simulink model "simRouteA_v4_11"  (R2015a)
settings: Solver=FixedStepDiscrete  StartTime=0.0  StopTime=36000  FixedStep=1  RelTol=1e-3
PreLoadFcn:
  | loadTimetable
StopFcn:
  | postProcess
undefined symbols (not defined in the file or in its folder): setBus1IntergenTime, setBus2IntergenTime, setBus3IntergenTime, setBus4IntergenTime
(part 7 of 7)

== system simRouteA_v4_11/atStopS18/calcPaxActivThisStop/Atomic Subsystem ==
  maxCap : Inport
  vacancy : Inport  Port=2
  paxAlight : Inport  Port=3
  paxArr : Inport  Port=4
  sec2Brd : Inport  Port=5
  Add : Sum
  Add1 : Sum
  Add2 : Sum
  Initial Value : InitialValue  Commented=on  InitialValue=0
  Min1 : MinMax  Inputs=2
  Min2 : MinMax  Inputs=2
  Product : Product
  Signal Latch : SignalLatch  Commented=on  MemoryWriteEdgeOption=Either  MemoryReadEdgeOption=Either  SpecifyReadEventPriority=on
      settings: InputPortMap=u0,u1,u2  OutputPortMap=o2
  Subtract : Sum  Inputs=+-
  Subtract1 : Sum  Inputs=-+
  Subtract2 : Sum  Inputs=+-
  Unit Delay : UnitDelay  SampleTime=-1
  newVacancy : Outport
  paxBoard : Outport  Port=2
  paxRemain : Outport  Port=3
  paxWait : Outport  Port=4
  dwellTime : Outport  Port=5
  corrPaxAlight : Outport  Port=6
  wires:
  Add/1 -> Min1/1, Subtract/1
  Min1/1 -> Subtract1/1, Subtract/2, Add2/1, paxBoard/1
  paxArr/1 -> Add1/1
  Add1/1 -> paxWait/1, Subtract1/2, Min1/2
  Subtract1/1 -> Unit Delay/1, paxRemain/1
  Unit Delay/1 -> Add1/2
  vacancy/1 -> Subtract2/2, Add/1
  maxCap/1 -> Subtract2/1
  Subtract/1 -> newVacancy/1
  Add2/1 -> Product/1
  sec2Brd/1 -> Product/2
  Product/1 -> dwellTime/1
  Subtract2/1 -> Min2/1
  Min2/1 -> corrPaxAlight/1, Add2/2, Add/2
  paxAlight/1 -> Min2/2

== system simRouteA_v4_11/atStopS18/calcPaxActivThisStop/calcPaxAlightS1 ==
  integrPax : Inport
  Subtract : Sum  Inputs=+-
  Unit Delay : UnitDelay  SampleTime=-1
  truPax : Outport
  intgPax : Outport  Port=2
  wires:
  integrPax/1 -> Unit Delay/1, intgPax/1, Subtract/1
  Subtract/1 -> truPax/1
  Unit Delay/1 -> Subtract/2

== system simRouteA_v4_11/atStopS18/calcPaxActivThisStop/calcPaxArrS1 ==
  integrPax : Inport
  Subtract : Sum  Inputs=+-
  Unit Delay : UnitDelay  SampleTime=-1
  truPax : Outport
  intgPax : Outport  Port=2
  wires:
  integrPax/1 -> Unit Delay/1, intgPax/1, Subtract/1
  Subtract/1 -> truPax/1
  Unit Delay/1 -> Subtract/2

== system simRouteA_v4_11/atStopS18/integrPaxAlightS1/Atomic Subsystem1 ==
  In1 : Inport
  Add : Sum
  Unit Delay : UnitDelay  SampleTime=-1
  Out1 : Outport
  wires:
  In1/1 -> Add/1
  Add/1 -> Out1/1, Unit Delay/1
  Unit Delay/1 -> Add/2

== system simRouteA_v4_11/atStopS18/integrPaxArrS1/Atomic Subsystem1 ==
  In1 : Inport
  Add : Sum
  Unit Delay : UnitDelay  SampleTime=-1
  Out1 : Outport
  wires:
  In1/1 -> Add/1
  Add/1 -> Out1/1, Unit Delay/1
  Unit Delay/1 -> Add/2

== system simRouteA_v4_11/atStopS2/busDwellThisStop/Subsystem2 ==
  dwellTime : Inport
  tStartSrvPax : Inport  Port=2
  Add1 : Sum
  Add2 : Sum
  Subtract : Sum  Inputs=+-
  Subtract1 : Sum  Inputs=+-
  Switch : Switch  Criteria=u2 > Threshold
  Unit Delay : UnitDelay  SampleTime=-1
  headWay : Constant  Value=3
  dwellTimeNew : Outport
  wires:
  Subtract/1 -> Switch/2
  Switch/1 -> Subtract1/1, Unit Delay/1
  headWay/1 -> Add2/1
  tStartSrvPax/1 -> Subtract1/2, Add1/2
  Add2/1 -> Switch/3
  dwellTime/1 -> Add1/1
  Subtract1/1 -> dwellTimeNew/1
  Add1/1 -> Switch/1, Subtract/1
  Unit Delay/1 -> Add2/2, Subtract/2

== system simRouteA_v4_11/atStopS2/calcPaxActivThisStop/Atomic Subsystem ==
  maxCap : Inport
  vacancy : Inport  Port=2
  paxAlight : Inport  Port=3
  paxArr : Inport  Port=4
  sec2Brd : Inport  Port=5
  Add : Sum
  Add1 : Sum
  Add2 : Sum
  Initial Value : InitialValue  Commented=on  InitialValue=0
  Min1 : MinMax  Inputs=2
  Min2 : MinMax  Inputs=2
  Product : Product
  Signal Latch : SignalLatch  Commented=on  MemoryWriteEdgeOption=Either  MemoryReadEdgeOption=Either  SpecifyReadEventPriority=on
      settings: InputPortMap=u0,u1,u2  OutputPortMap=o2
  Subtract : Sum  Inputs=+-
  Subtract1 : Sum  Inputs=-+
  Subtract2 : Sum  Inputs=+-
  Unit Delay : UnitDelay  SampleTime=-1
  newVacancy : Outport
  paxBoard : Outport  Port=2
  paxRemain : Outport  Port=3
  paxWait : Outport  Port=4
  dwellTime : Outport  Port=5
  corrPaxAlight : Outport  Port=6
  wires:
  Add/1 -> Min1/1, Subtract/1
  Min1/1 -> Subtract1/1, Subtract/2, Add2/1, paxBoard/1
  paxArr/1 -> Add1/1
  Add1/1 -> paxWait/1, Subtract1/2, Min1/2
  Subtract1/1 -> Unit Delay/1, paxRemain/1
  Unit Delay/1 -> Add1/2
  vacancy/1 -> Subtract2/2, Add/1
  maxCap/1 -> Subtract2/1
  Subtract/1 -> newVacancy/1
  Add2/1 -> Product/1
  sec2Brd/1 -> Product/2
  Product/1 -> dwellTime/1
  Subtract2/1 -> Min2/1
  Min2/1 -> corrPaxAlight/1, Add2/2, Add/2
  paxAlight/1 -> Min2/2

== system simRouteA_v4_11/atStopS2/calcPaxActivThisStop/calcPaxAlightS1 ==
  integrPax : Inport
  Subtract : Sum  Inputs=+-
  Unit Delay : UnitDelay  SampleTime=-1
  truPax : Outport
  intgPax : Outport  Port=2
  wires:
  integrPax/1 -> Unit Delay/1, intgPax/1, Subtract/1
  Subtract/1 -> truPax/1
  Unit Delay/1 -> Subtract/2

== system simRouteA_v4_11/atStopS2/calcPaxActivThisStop/calcPaxArrS1 ==
  integrPax : Inport
  Subtract : Sum  Inputs=+-
  Unit Delay : UnitDelay  SampleTime=-1
  truPax : Outport
  intgPax : Outport  Port=2
  wires:
  integrPax/1 -> Unit Delay/1, intgPax/1, Subtract/1
  Subtract/1 -> truPax/1
  Unit Delay/1 -> Subtract/2

== system simRouteA_v4_11/atStopS2/integrPaxAlightS1/Atomic Subsystem1 ==
  In1 : Inport
  Add : Sum
  Unit Delay : UnitDelay  SampleTime=-1
  Out1 : Outport
  wires:
  In1/1 -> Add/1
  Add/1 -> Out1/1, Unit Delay/1
  Unit Delay/1 -> Add/2

== system simRouteA_v4_11/atStopS2/integrPaxArrS1/Atomic Subsystem1 ==
  In1 : Inport
  Add : Sum
  Unit Delay : UnitDelay  SampleTime=-1
  Out1 : Outport
  wires:
  In1/1 -> Add/1
  Add/1 -> Out1/1, Unit Delay/1
  Unit Delay/1 -> Add/2

== system simRouteA_v4_11/atStopS3/busDwellThisStop/Subsystem2 ==
  dwellTime : Inport
  tStartSrvPax : Inport  Port=2
  Add1 : Sum
  Add2 : Sum
  Subtract : Sum  Inputs=+-
  Subtract1 : Sum  Inputs=+-
  Switch : Switch  Criteria=u2 > Threshold
  Unit Delay : UnitDelay  SampleTime=-1
  headWay : Constant  Value=3
  dwellTimeNew : Outport
  wires:
  Subtract/1 -> Switch/2
  Switch/1 -> Subtract1/1, Unit Delay/1
  headWay/1 -> Add2/1
  tStartSrvPax/1 -> Subtract1/2, Add1/2
  Add2/1 -> Switch/3
  dwellTime/1 -> Add1/1
  Subtract1/1 -> dwellTimeNew/1
  Add1/1 -> Switch/1, Subtract/1
  Unit Delay/1 -> Add2/2, Subtract/2

== system simRouteA_v4_11/atStopS3/calcPaxActivThisStop/Atomic Subsystem ==
  maxCap : Inport
  vacancy : Inport  Port=2
  paxAlight : Inport  Port=3
  paxArr : Inport  Port=4
  sec2Brd : Inport  Port=5
  Add : Sum
  Add1 : Sum
  Add2 : Sum
  Initial Value : InitialValue  Commented=on  InitialValue=0
  Min1 : MinMax  Inputs=2
  Min2 : MinMax  Inputs=2
  Product : Product
  Signal Latch : SignalLatch  Commented=on  MemoryWriteEdgeOption=Either  MemoryReadEdgeOption=Either  SpecifyReadEventPriority=on
      settings: InputPortMap=u0,u1,u2  OutputPortMap=o2
  Subtract : Sum  Inputs=+-
  Subtract1 : Sum  Inputs=-+
  Subtract2 : Sum  Inputs=+-
  Unit Delay : UnitDelay  SampleTime=-1
  newVacancy : Outport
  paxBoard : Outport  Port=2
  paxRemain : Outport  Port=3
  paxWait : Outport  Port=4
  dwellTime : Outport  Port=5
  corrPaxAlight : Outport  Port=6
  wires:
  Add/1 -> Min1/1, Subtract/1
  Min1/1 -> Subtract1/1, Subtract/2, Add2/1, paxBoard/1
  paxArr/1 -> Add1/1
  Add1/1 -> paxWait/1, Subtract1/2, Min1/2
  Subtract1/1 -> Unit Delay/1, paxRemain/1
  Unit Delay/1 -> Add1/2
  vacancy/1 -> Subtract2/2, Add/1
  maxCap/1 -> Subtract2/1
  Subtract/1 -> newVacancy/1
  Add2/1 -> Product/1
  sec2Brd/1 -> Product/2
  Product/1 -> dwellTime/1
  Subtract2/1 -> Min2/1
  Min2/1 -> corrPaxAlight/1, Add2/2, Add/2
  paxAlight/1 -> Min2/2

== system simRouteA_v4_11/atStopS3/calcPaxActivThisStop/calcPaxAlightS1 ==
  integrPax : Inport
  Subtract : Sum  Inputs=+-
  Unit Delay : UnitDelay  SampleTime=-1
  truPax : Outport
  intgPax : Outport  Port=2
  wires:
  integrPax/1 -> Unit Delay/1, intgPax/1, Subtract/1
  Subtract/1 -> truPax/1
  Unit Delay/1 -> Subtract/2

== system simRouteA_v4_11/atStopS3/calcPaxActivThisStop/calcPaxArrS1 ==
  integrPax : Inport
  Subtract : Sum  Inputs=+-
  Unit Delay : UnitDelay  SampleTime=-1
  truPax : Outport
  intgPax : Outport  Port=2
  wires:
  integrPax/1 -> Unit Delay/1, intgPax/1, Subtract/1
  Subtract/1 -> truPax/1
  Unit Delay/1 -> Subtract/2

== system simRouteA_v4_11/atStopS3/integrPaxAlightS1/Atomic Subsystem1 ==
  In1 : Inport
  Add : Sum
  Unit Delay : UnitDelay  SampleTime=-1
  Out1 : Outport
  wires:
  In1/1 -> Add/1
  Add/1 -> Out1/1, Unit Delay/1
  Unit Delay/1 -> Add/2

== system simRouteA_v4_11/atStopS3/integrPaxArrS1/Atomic Subsystem1 ==
  In1 : Inport
  Add : Sum
  Unit Delay : UnitDelay  SampleTime=-1
  Out1 : Outport
  wires:
  In1/1 -> Add/1
  Add/1 -> Out1/1, Unit Delay/1
  Unit Delay/1 -> Add/2

== system simRouteA_v4_11/atStopS4/busDwellThisStop/Subsystem2 ==
  dwellTime : Inport
  tStartSrvPax : Inport  Port=2
  Add1 : Sum
  Add2 : Sum
  Subtract : Sum  Inputs=+-
  Subtract1 : Sum  Inputs=+-
  Switch : Switch  Criteria=u2 > Threshold
  Unit Delay : UnitDelay  SampleTime=-1
  headWay : Constant  Value=3
  dwellTimeNew : Outport
  wires:
  Subtract/1 -> Switch/2
  Switch/1 -> Subtract1/1, Unit Delay/1
  headWay/1 -> Add2/1
  tStartSrvPax/1 -> Subtract1/2, Add1/2
  Add2/1 -> Switch/3
  dwellTime/1 -> Add1/1
  Subtract1/1 -> dwellTimeNew/1
  Add1/1 -> Switch/1, Subtract/1
  Unit Delay/1 -> Add2/2, Subtract/2

== system simRouteA_v4_11/atStopS4/calcPaxActivThisStop/Atomic Subsystem ==
  maxCap : Inport
  vacancy : Inport  Port=2
  paxAlight : Inport  Port=3
  paxArr : Inport  Port=4
  sec2Brd : Inport  Port=5
  Add : Sum
  Add1 : Sum
  Add2 : Sum
  Initial Value : InitialValue  Commented=on  InitialValue=0
  Min1 : MinMax  Inputs=2
  Min2 : MinMax  Inputs=2
  Product : Product
  Signal Latch : SignalLatch  Commented=on  MemoryWriteEdgeOption=Either  MemoryReadEdgeOption=Either  SpecifyReadEventPriority=on
      settings: InputPortMap=u0,u1,u2  OutputPortMap=o2
  Subtract : Sum  Inputs=+-
  Subtract1 : Sum  Inputs=-+
  Subtract2 : Sum  Inputs=+-
  Unit Delay : UnitDelay  SampleTime=-1
  newVacancy : Outport
  paxBoard : Outport  Port=2
  paxRemain : Outport  Port=3
  paxWait : Outport  Port=4
  dwellTime : Outport  Port=5
  corrPaxAlight : Outport  Port=6
  wires:
  Add/1 -> Min1/1, Subtract/1
  Min1/1 -> Subtract1/1, Subtract/2, Add2/1, paxBoard/1
  paxArr/1 -> Add1/1
  Add1/1 -> paxWait/1, Subtract1/2, Min1/2
  Subtract1/1 -> Unit Delay/1, paxRemain/1
  Unit Delay/1 -> Add1/2
  vacancy/1 -> Subtract2/2, Add/1
  maxCap/1 -> Subtract2/1
  Subtract/1 -> newVacancy/1
  Add2/1 -> Product/1
  sec2Brd/1 -> Product/2
  Product/1 -> dwellTime/1
  Subtract2/1 -> Min2/1
  Min2/1 -> corrPaxAlight/1, Add2/2, Add/2
  paxAlight/1 -> Min2/2

== system simRouteA_v4_11/atStopS4/calcPaxActivThisStop/calcPaxAlightS1 ==
  integrPax : Inport
  Subtract : Sum  Inputs=+-
  Unit Delay : UnitDelay  SampleTime=-1
  truPax : Outport
  intgPax : Outport  Port=2
  wires:
  integrPax/1 -> Unit Delay/1, intgPax/1, Subtract/1
  Subtract/1 -> truPax/1
  Unit Delay/1 -> Subtract/2

== system simRouteA_v4_11/atStopS4/calcPaxActivThisStop/calcPaxArrS1 ==
  integrPax : Inport
  Subtract : Sum  Inputs=+-
  Unit Delay : UnitDelay  SampleTime=-1
  truPax : Outport
  intgPax : Outport  Port=2
  wires:
  integrPax/1 -> Unit Delay/1, intgPax/1, Subtract/1
  Subtract/1 -> truPax/1
  Unit Delay/1 -> Subtract/2

== system simRouteA_v4_11/atStopS4/integrPaxAlightS1/Atomic Subsystem1 ==
  In1 : Inport
  Add : Sum
  Unit Delay : UnitDelay  SampleTime=-1
  Out1 : Outport
  wires:
  In1/1 -> Add/1
  Add/1 -> Out1/1, Unit Delay/1
  Unit Delay/1 -> Add/2

== system simRouteA_v4_11/atStopS4/integrPaxArrS1/Atomic Subsystem1 ==
  In1 : Inport
  Add : Sum
  Unit Delay : UnitDelay  SampleTime=-1
  Out1 : Outport
  wires:
  In1/1 -> Add/1
  Add/1 -> Out1/1, Unit Delay/1
  Unit Delay/1 -> Add/2

== system simRouteA_v4_11/atStopS5/busDwellThisStop/Subsystem2 ==
  dwellTime : Inport
  tStartSrvPax : Inport  Port=2
  Add1 : Sum
  Add2 : Sum
  Subtract : Sum  Inputs=+-
  Subtract1 : Sum  Inputs=+-
  Switch : Switch  Criteria=u2 > Threshold
  Unit Delay : UnitDelay  SampleTime=-1
  headWay : Constant  Value=3
  dwellTimeNew : Outport
  wires:
  Subtract/1 -> Switch/2
  Switch/1 -> Subtract1/1, Unit Delay/1
  headWay/1 -> Add2/1
  tStartSrvPax/1 -> Subtract1/2, Add1/2
  Add2/1 -> Switch/3
  dwellTime/1 -> Add1/1
  Subtract1/1 -> dwellTimeNew/1
  Add1/1 -> Switch/1, Subtract/1
  Unit Delay/1 -> Add2/2, Subtract/2

== system simRouteA_v4_11/atStopS5/calcPaxActivThisStop/Atomic Subsystem ==
  maxCap : Inport
  vacancy : Inport  Port=2
  paxAlight : Inport  Port=3
  paxArr : Inport  Port=4
  sec2Brd : Inport  Port=5
  Add : Sum
  Add1 : Sum
  Add2 : Sum
  Initial Value : InitialValue  Commented=on  InitialValue=0
  Min1 : MinMax  Inputs=2
  Min2 : MinMax  Inputs=2
  Product : Product
  Signal Latch : SignalLatch  Commented=on  MemoryWriteEdgeOption=Either  MemoryReadEdgeOption=Either  SpecifyReadEventPriority=on
      settings: InputPortMap=u0,u1,u2  OutputPortMap=o2
  Subtract : Sum  Inputs=+-
  Subtract1 : Sum  Inputs=-+
  Subtract2 : Sum  Inputs=+-
  Unit Delay : UnitDelay  SampleTime=-1
  newVacancy : Outport
  paxBoard : Outport  Port=2
  paxRemain : Outport  Port=3
  paxWait : Outport  Port=4
  dwellTime : Outport  Port=5
  corrPaxAlight : Outport  Port=6
  wires:
  Add/1 -> Min1/1, Subtract/1
  Min1/1 -> Subtract1/1, Subtract/2, Add2/1, paxBoard/1
  paxArr/1 -> Add1/1
  Add1/1 -> paxWait/1, Subtract1/2, Min1/2
  Subtract1/1 -> Unit Delay/1, paxRemain/1
  Unit Delay/1 -> Add1/2
  vacancy/1 -> Subtract2/2, Add/1
  maxCap/1 -> Subtract2/1
  Subtract/1 -> newVacancy/1
  Add2/1 -> Product/1
  sec2Brd/1 -> Product/2
  Product/1 -> dwellTime/1
  Subtract2/1 -> Min2/1
  Min2/1 -> corrPaxAlight/1, Add2/2, Add/2
  paxAlight/1 -> Min2/2

== system simRouteA_v4_11/atStopS5/calcPaxActivThisStop/calcPaxAlightS1 ==
  integrPax : Inport
  Subtract : Sum  Inputs=+-
  Unit Delay : UnitDelay  SampleTime=-1
  truPax : Outport
  intgPax : Outport  Port=2
  wires:
  integrPax/1 -> Unit Delay/1, intgPax/1, Subtract/1
  Subtract/1 -> truPax/1
  Unit Delay/1 -> Subtract/2

== system simRouteA_v4_11/atStopS5/calcPaxActivThisStop/calcPaxArrS1 ==
  integrPax : Inport
  Subtract : Sum  Inputs=+-
  Unit Delay : UnitDelay  SampleTime=-1
  truPax : Outport
  intgPax : Outport  Port=2
  wires:
  integrPax/1 -> Unit Delay/1, intgPax/1, Subtract/1
  Subtract/1 -> truPax/1
  Unit Delay/1 -> Subtract/2

== system simRouteA_v4_11/atStopS5/integrPaxAlightS1/Atomic Subsystem1 ==
  In1 : Inport
  Add : Sum
  Unit Delay : UnitDelay  SampleTime=-1
  Out1 : Outport
  wires:
  In1/1 -> Add/1
  Add/1 -> Out1/1, Unit Delay/1
  Unit Delay/1 -> Add/2

== system simRouteA_v4_11/atStopS5/integrPaxArrS1/Atomic Subsystem1 ==
  In1 : Inport
  Add : Sum
  Unit Delay : UnitDelay  SampleTime=-1
  Out1 : Outport
  wires:
  In1/1 -> Add/1
  Add/1 -> Out1/1, Unit Delay/1
  Unit Delay/1 -> Add/2

== system simRouteA_v4_11/atStopS6/busDwellThisStop/Subsystem2 ==
  dwellTime : Inport
  tStartSrvPax : Inport  Port=2
  Add1 : Sum
  Add2 : Sum
  Subtract : Sum  Inputs=+-
  Subtract1 : Sum  Inputs=+-
  Switch : Switch  Criteria=u2 > Threshold
  Unit Delay : UnitDelay  SampleTime=-1
  headWay : Constant  Value=3
  dwellTimeNew : Outport
  wires:
  Subtract/1 -> Switch/2
  Switch/1 -> Subtract1/1, Unit Delay/1
  headWay/1 -> Add2/1
  tStartSrvPax/1 -> Subtract1/2, Add1/2
  Add2/1 -> Switch/3
  dwellTime/1 -> Add1/1
  Subtract1/1 -> dwellTimeNew/1
  Add1/1 -> Switch/1, Subtract/1
  Unit Delay/1 -> Add2/2, Subtract/2

== system simRouteA_v4_11/atStopS6/calcPaxActivThisStop/Atomic Subsystem ==
  maxCap : Inport
  vacancy : Inport  Port=2
  paxAlight : Inport  Port=3
  paxArr : Inport  Port=4
  sec2Brd : Inport  Port=5
  Add : Sum
  Add1 : Sum
  Add2 : Sum
  Initial Value : InitialValue  Commented=on  InitialValue=0
  Min1 : MinMax  Inputs=2
  Min2 : MinMax  Inputs=2
  Product : Product
  Signal Latch : SignalLatch  Commented=on  MemoryWriteEdgeOption=Either  MemoryReadEdgeOption=Either  SpecifyReadEventPriority=on
      settings: InputPortMap=u0,u1,u2  OutputPortMap=o2
  Subtract : Sum  Inputs=+-
  Subtract1 : Sum  Inputs=-+
  Subtract2 : Sum  Inputs=+-
  Unit Delay : UnitDelay  SampleTime=-1
  newVacancy : Outport
  paxBoard : Outport  Port=2
  paxRemain : Outport  Port=3
  paxWait : Outport  Port=4
  dwellTime : Outport  Port=5
  corrPaxAlight : Outport  Port=6
  wires:
  Add/1 -> Min1/1, Subtract/1
  Min1/1 -> Subtract1/1, Subtract/2, Add2/1, paxBoard/1
  paxArr/1 -> Add1/1
  Add1/1 -> paxWait/1, Subtract1/2, Min1/2
  Subtract1/1 -> Unit Delay/1, paxRemain/1
  Unit Delay/1 -> Add1/2
  vacancy/1 -> Subtract2/2, Add/1
  maxCap/1 -> Subtract2/1
  Subtract/1 -> newVacancy/1
  Add2/1 -> Product/1
  sec2Brd/1 -> Product/2
  Product/1 -> dwellTime/1
  Subtract2/1 -> Min2/1
  Min2/1 -> corrPaxAlight/1, Add2/2, Add/2
  paxAlight/1 -> Min2/2

== system simRouteA_v4_11/atStopS6/calcPaxActivThisStop/calcPaxAlightS1 ==
  integrPax : Inport
  Subtract : Sum  Inputs=+-
  Unit Delay : UnitDelay  SampleTime=-1
  truPax : Outport
  intgPax : Outport  Port=2
  wires:
  integrPax/1 -> Unit Delay/1, intgPax/1, Subtract/1
  Subtract/1 -> truPax/1
  Unit Delay/1 -> Subtract/2

== system simRouteA_v4_11/atStopS6/calcPaxActivThisStop/calcPaxArrS1 ==
  integrPax : Inport
  Subtract : Sum  Inputs=+-
  Unit Delay : UnitDelay  SampleTime=-1
  truPax : Outport
  intgPax : Outport  Port=2
  wires:
  integrPax/1 -> Unit Delay/1, intgPax/1, Subtract/1
  Subtract/1 -> truPax/1
  Unit Delay/1 -> Subtract/2

== system simRouteA_v4_11/atStopS6/integrPaxAlightS1/Atomic Subsystem1 ==
  In1 : Inport
  Add : Sum
  Unit Delay : UnitDelay  SampleTime=-1
  Out1 : Outport
  wires:
  In1/1 -> Add/1
  Add/1 -> Out1/1, Unit Delay/1
  Unit Delay/1 -> Add/2

== system simRouteA_v4_11/atStopS6/integrPaxArrS1/Atomic Subsystem1 ==
  In1 : Inport
  Add : Sum
  Unit Delay : UnitDelay  SampleTime=-1
  Out1 : Outport
  wires:
  In1/1 -> Add/1
  Add/1 -> Out1/1, Unit Delay/1
  Unit Delay/1 -> Add/2

== system simRouteA_v4_11/atStopS7/busDwellThisStop/Subsystem2 ==
  dwellTime : Inport
  tStartSrvPax : Inport  Port=2
  Add1 : Sum
  Add2 : Sum
  Subtract : Sum  Inputs=+-
  Subtract1 : Sum  Inputs=+-
  Switch : Switch  Criteria=u2 > Threshold
  Unit Delay : UnitDelay  SampleTime=-1
  headWay : Constant  Value=3
  dwellTimeNew : Outport
  wires:
  Subtract/1 -> Switch/2
  Switch/1 -> Subtract1/1, Unit Delay/1
  headWay/1 -> Add2/1
  tStartSrvPax/1 -> Subtract1/2, Add1/2
  Add2/1 -> Switch/3
  dwellTime/1 -> Add1/1
  Subtract1/1 -> dwellTimeNew/1
  Add1/1 -> Switch/1, Subtract/1
  Unit Delay/1 -> Add2/2, Subtract/2

== system simRouteA_v4_11/atStopS7/calcPaxActivThisStop/Atomic Subsystem ==
  maxCap : Inport
  vacancy : Inport  Port=2
  paxAlight : Inport  Port=3
  paxArr : Inport  Port=4
  sec2Brd : Inport  Port=5
  Add : Sum
  Add1 : Sum
  Add2 : Sum
  Initial Value : InitialValue  Commented=on  InitialValue=0
  Min1 : MinMax  Inputs=2
  Min2 : MinMax  Inputs=2
  Product : Product
  Signal Latch : SignalLatch  Commented=on  MemoryWriteEdgeOption=Either  MemoryReadEdgeOption=Either  SpecifyReadEventPriority=on
      settings: InputPortMap=u0,u1,u2  OutputPortMap=o2
  Subtract : Sum  Inputs=+-
  Subtract1 : Sum  Inputs=-+
  Subtract2 : Sum  Inputs=+-
  Unit Delay : UnitDelay  SampleTime=-1
  newVacancy : Outport
  paxBoard : Outport  Port=2
  paxRemain : Outport  Port=3
  paxWait : Outport  Port=4
  dwellTime : Outport  Port=5
  corrPaxAlight : Outport  Port=6
  wires:
  Add/1 -> Min1/1, Subtract/1
  Min1/1 -> Subtract1/1, Subtract/2, Add2/1, paxBoard/1
  paxArr/1 -> Add1/1
  Add1/1 -> paxWait/1, Subtract1/2, Min1/2
  Subtract1/1 -> Unit Delay/1, paxRemain/1
  Unit Delay/1 -> Add1/2
  vacancy/1 -> Subtract2/2, Add/1
  maxCap/1 -> Subtract2/1
  Subtract/1 -> newVacancy/1
  Add2/1 -> Product/1
  sec2Brd/1 -> Product/2
  Product/1 -> dwellTime/1
  Subtract2/1 -> Min2/1
  Min2/1 -> corrPaxAlight/1, Add2/2, Add/2
  paxAlight/1 -> Min2/2

== system simRouteA_v4_11/atStopS7/calcPaxActivThisStop/calcPaxAlightS1 ==
  integrPax : Inport
  Subtract : Sum  Inputs=+-
  Unit Delay : UnitDelay  SampleTime=-1
  truPax : Outport
  intgPax : Outport  Port=2
  wires:
  integrPax/1 -> Unit Delay/1, intgPax/1, Subtract/1
  Subtract/1 -> truPax/1
  Unit Delay/1 -> Subtract/2

== system simRouteA_v4_11/atStopS7/calcPaxActivThisStop/calcPaxArrS1 ==
  integrPax : Inport
  Subtract : Sum  Inputs=+-
  Unit Delay : UnitDelay  SampleTime=-1
  truPax : Outport
  intgPax : Outport  Port=2
  wires:
  integrPax/1 -> Unit Delay/1, intgPax/1, Subtract/1
  Subtract/1 -> truPax/1
  Unit Delay/1 -> Subtract/2

== system simRouteA_v4_11/atStopS7/integrPaxAlightS1/Atomic Subsystem1 ==
  In1 : Inport
  Add : Sum
  Unit Delay : UnitDelay  SampleTime=-1
  Out1 : Outport
  wires:
  In1/1 -> Add/1
  Add/1 -> Out1/1, Unit Delay/1
  Unit Delay/1 -> Add/2

== system simRouteA_v4_11/atStopS7/integrPaxArrS1/Atomic Subsystem1 ==
  In1 : Inport
  Add : Sum
  Unit Delay : UnitDelay  SampleTime=-1
  Out1 : Outport
  wires:
  In1/1 -> Add/1
  Add/1 -> Out1/1, Unit Delay/1
  Unit Delay/1 -> Add/2

== system simRouteA_v4_11/atStopS8/busDwellThisStop/Subsystem2 ==
  dwellTime : Inport
  tStartSrvPax : Inport  Port=2
  Add1 : Sum
  Add2 : Sum
  Subtract : Sum  Inputs=+-
  Subtract1 : Sum  Inputs=+-
  Switch : Switch  Criteria=u2 > Threshold
  Unit Delay : UnitDelay  SampleTime=-1
  headWay : Constant  Value=3
  dwellTimeNew : Outport
  wires:
  Subtract/1 -> Switch/2
  Switch/1 -> Subtract1/1, Unit Delay/1
  headWay/1 -> Add2/1
  tStartSrvPax/1 -> Subtract1/2, Add1/2
  Add2/1 -> Switch/3
  dwellTime/1 -> Add1/1
  Subtract1/1 -> dwellTimeNew/1
  Add1/1 -> Switch/1, Subtract/1
  Unit Delay/1 -> Add2/2, Subtract/2

== system simRouteA_v4_11/atStopS8/calcPaxActivThisStop/Atomic Subsystem ==
  maxCap : Inport
  vacancy : Inport  Port=2
  paxAlight : Inport  Port=3
  paxArr : Inport  Port=4
  sec2Brd : Inport  Port=5
  Add : Sum
  Add1 : Sum
  Add2 : Sum
  Initial Value : InitialValue  Commented=on  InitialValue=0
  Min1 : MinMax  Inputs=2
  Min2 : MinMax  Inputs=2
  Product : Product
  Signal Latch : SignalLatch  Commented=on  MemoryWriteEdgeOption=Either  MemoryReadEdgeOption=Either  SpecifyReadEventPriority=on
      settings: InputPortMap=u0,u1,u2  OutputPortMap=o2
  Subtract : Sum  Inputs=+-
  Subtract1 : Sum  Inputs=-+
  Subtract2 : Sum  Inputs=+-
  Unit Delay : UnitDelay  SampleTime=-1
  newVacancy : Outport
  paxBoard : Outport  Port=2
  paxRemain : Outport  Port=3
  paxWait : Outport  Port=4
  dwellTime : Outport  Port=5
  corrPaxAlight : Outport  Port=6
  wires:
  Add/1 -> Min1/1, Subtract/1
  Min1/1 -> Subtract1/1, Subtract/2, Add2/1, paxBoard/1
  paxArr/1 -> Add1/1
  Add1/1 -> paxWait/1, Subtract1/2, Min1/2
  Subtract1/1 -> Unit Delay/1, paxRemain/1
  Unit Delay/1 -> Add1/2
  vacancy/1 -> Subtract2/2, Add/1
  maxCap/1 -> Subtract2/1
  Subtract/1 -> newVacancy/1
  Add2/1 -> Product/1
  sec2Brd/1 -> Product/2
  Product/1 -> dwellTime/1
  Subtract2/1 -> Min2/1
  Min2/1 -> corrPaxAlight/1, Add2/2, Add/2
  paxAlight/1 -> Min2/2

== system simRouteA_v4_11/atStopS8/calcPaxActivThisStop/calcPaxAlightS1 ==
  integrPax : Inport
  Subtract : Sum  Inputs=+-
  Unit Delay : UnitDelay  SampleTime=-1
  truPax : Outport
  intgPax : Outport  Port=2
  wires:
  integrPax/1 -> Unit Delay/1, intgPax/1, Subtract/1
  Subtract/1 -> truPax/1
  Unit Delay/1 -> Subtract/2

== system simRouteA_v4_11/atStopS8/calcPaxActivThisStop/calcPaxArrS1 ==
  integrPax : Inport
  Subtract : Sum  Inputs=+-
  Unit Delay : UnitDelay  SampleTime=-1
  truPax : Outport
  intgPax : Outport  Port=2
  wires:
  integrPax/1 -> Unit Delay/1, intgPax/1, Subtract/1
  Subtract/1 -> truPax/1
  Unit Delay/1 -> Subtract/2

== system simRouteA_v4_11/atStopS8/integrPaxAlightS1/Atomic Subsystem1 ==
  In1 : Inport
  Add : Sum
  Unit Delay : UnitDelay  SampleTime=-1
  Out1 : Outport
  wires:
  In1/1 -> Add/1
  Add/1 -> Out1/1, Unit Delay/1
  Unit Delay/1 -> Add/2

== system simRouteA_v4_11/atStopS8/integrPaxArrS1/Atomic Subsystem1 ==
  In1 : Inport
  Add : Sum
  Unit Delay : UnitDelay  SampleTime=-1
  Out1 : Outport
  wires:
  In1/1 -> Add/1
  Add/1 -> Out1/1, Unit Delay/1
  Unit Delay/1 -> Add/2

== system simRouteA_v4_11/atStopS9/busDwellThisStop/Subsystem2 ==
  dwellTime : Inport
  tStartSrvPax : Inport  Port=2
  Add1 : Sum
  Add2 : Sum
  Subtract : Sum  Inputs=+-
  Subtract1 : Sum  Inputs=+-
  Switch : Switch  Criteria=u2 > Threshold
  Unit Delay : UnitDelay  SampleTime=-1
  headWay : Constant  Value=3
  dwellTimeNew : Outport
  wires:
  Subtract/1 -> Switch/2
  Switch/1 -> Subtract1/1, Unit Delay/1
  headWay/1 -> Add2/1
  tStartSrvPax/1 -> Subtract1/2, Add1/2
  Add2/1 -> Switch/3
  dwellTime/1 -> Add1/1
  Subtract1/1 -> dwellTimeNew/1
  Add1/1 -> Switch/1, Subtract/1
  Unit Delay/1 -> Add2/2, Subtract/2

== system simRouteA_v4_11/atStopS9/calcPaxActivThisStop/Atomic Subsystem ==
  maxCap : Inport
  vacancy : Inport  Port=2
  paxAlight : Inport  Port=3
  paxArr : Inport  Port=4
  sec2Brd : Inport  Port=5
  Add : Sum
  Add1 : Sum
  Add2 : Sum
  Initial Value : InitialValue  Commented=on  InitialValue=0
  Min1 : MinMax  Inputs=2
  Min2 : MinMax  Inputs=2
  Product : Product
  Signal Latch : SignalLatch  Commented=on  MemoryWriteEdgeOption=Either  MemoryReadEdgeOption=Either  SpecifyReadEventPriority=on
      settings: InputPortMap=u0,u1,u2  OutputPortMap=o2
  Subtract : Sum  Inputs=+-
  Subtract1 : Sum  Inputs=-+
  Subtract2 : Sum  Inputs=+-
  Unit Delay : UnitDelay  SampleTime=-1
  newVacancy : Outport
  paxBoard : Outport  Port=2
  paxRemain : Outport  Port=3
  paxWait : Outport  Port=4
  dwellTime : Outport  Port=5
  corrPaxAlight : Outport  Port=6
  wires:
  Add/1 -> Min1/1, Subtract/1
  Min1/1 -> Subtract1/1, Subtract/2, Add2/1, paxBoard/1
  paxArr/1 -> Add1/1
  Add1/1 -> paxWait/1, Subtract1/2, Min1/2
  Subtract1/1 -> Unit Delay/1, paxRemain/1
  Unit Delay/1 -> Add1/2
  vacancy/1 -> Subtract2/2, Add/1
  maxCap/1 -> Subtract2/1
  Subtract/1 -> newVacancy/1
  Add2/1 -> Product/1
  sec2Brd/1 -> Product/2
  Product/1 -> dwellTime/1
  Subtract2/1 -> Min2/1
  Min2/1 -> corrPaxAlight/1, Add2/2, Add/2
  paxAlight/1 -> Min2/2

== system simRouteA_v4_11/atStopS9/calcPaxActivThisStop/calcPaxAlightS1 ==
  integrPax : Inport
  Subtract : Sum  Inputs=+-
  Unit Delay : UnitDelay  SampleTime=-1
  truPax : Outport
  intgPax : Outport  Port=2
  wires:
  integrPax/1 -> Unit Delay/1, intgPax/1, Subtract/1
  Subtract/1 -> truPax/1
  Unit Delay/1 -> Subtract/2

== system simRouteA_v4_11/atStopS9/calcPaxActivThisStop/calcPaxArrS1 ==
  integrPax : Inport
  Subtract : Sum  Inputs=+-
  Unit Delay : UnitDelay  SampleTime=-1
  truPax : Outport
  intgPax : Outport  Port=2
  wires:
  integrPax/1 -> Unit Delay/1, intgPax/1, Subtract/1
  Subtract/1 -> truPax/1
  Unit Delay/1 -> Subtract/2

== system simRouteA_v4_11/atStopS9/integrPaxAlightS1/Atomic Subsystem1 ==
  In1 : Inport
  Add : Sum
  Unit Delay : UnitDelay  SampleTime=-1
  Out1 : Outport
  wires:
  In1/1 -> Add/1
  Add/1 -> Out1/1, Unit Delay/1
  Unit Delay/1 -> Add/2

== system simRouteA_v4_11/atStopS9/integrPaxArrS1/Atomic Subsystem1 ==
  In1 : Inport
  Add : Sum
  Unit Delay : UnitDelay  SampleTime=-1
  Out1 : Outport
  wires:
  In1/1 -> Add/1
  Add/1 -> Out1/1, Unit Delay/1
  Unit Delay/1 -> Add/2
